simulink model "Test_filter"  (Simulink 7.6)
settings: Solver=ode45  StartTime=0.0  StopTime=10.0  RelTol=1e-3
libraries: simulink x3
settings Model: Creator=administrator  LastModifiedBy=administrator

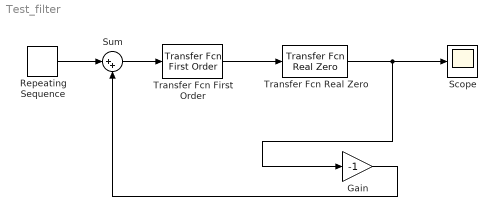
== system Test_filter ==
  Gain : Gain  Gain=-1
  Repeating Sequence : simulink/Sources/Repeating Sequence  SystemSampleTime=-1  rep_seq_t="[     0    0.0100    0.0200    0.0300    0.0400    0.0500    0.0600    0.0700    0.0800    0.0900    0.1000    0.1100    0.1200    0.1300    0.1400    0.1500]"  rep_seq_y="[    1.0000    0.5000    0.2500    0.1250    0.0625    0.0312    0.0156    0.0078    0.0039    0.0020    0.0010    0.0005    0.0002    0.0001    0.0001    0.0000]"
  Scope : Scope
  Sum : Sum  Inputs=|++
  Transfer Fcn First Order : simulink/Discrete/Transfer Fcn First Order  SystemSampleTime=-1  PoleZ=0.95  ICPrevOutput=0.0  DoSatur=off
  Transfer Fcn Real Zero : simulink/Discrete/Transfer Fcn Real Zero  SystemSampleTime=-1  ZeroZ=0.5  ICPrevInput=0.0  DoSatur=off
  wires:
  Transfer Fcn First Order/1 -> Transfer Fcn Real Zero/1
  Sum/1 -> Transfer Fcn First Order/1
  Repeating Sequence/1 -> Sum/1
  Transfer Fcn Real Zero/1 -> Scope/1, Gain/1
  Gain/1 -> Sum/2
